simulink model "ssbdemof"  (Simulink 4.00)
settings: Solver=FixedStepDiscrete  SolverMode=SingleTasking  StartTime=0.0  StopTime=99999999  RelTol=1e-3  AbsTol=1e-6
libraries: dspsnks3 x2, dspsrcs3 x2, simulink3 x2, dspxfrm3 x1, dspindex x1
settings Model: CovMetricSettings=d  Creator=don  LastModifiedBy=asharma  SaveTime=off  SaveOutput=off  LimitDataPoints=off  IntegerOverflowMsg=none  RTWOptions=-aRollThreshold=2  ExtModeTrigMode=oneshot  ExtModeArmWhenConnect=off  BlockReductionOpt=off

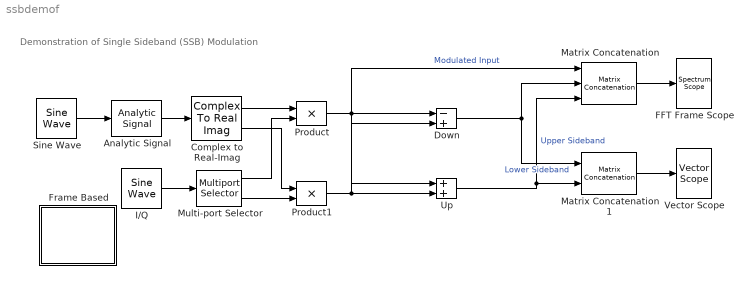
== system ssbdemof ==
  note: Demonstration of
      | Single Sideband (SSB)
      | Modulation
  Analytic Signal : dspxfrm3/Analytic Signal  N=100
  Complex to Real-Imag : ComplexToRealImag  Output=RealAndImag
  Down : Sum  Inputs=-+  SaturateOnIntegerOverflow=on
  FFT Frame Scope : dspsnks3/Spectrum Scope  ScopeProperties=on  Domain=Frequency  HorizSpan=1  UseBuffer=off  BufferSize=128  Overlap=64  inpFftLenInherit=off  FFTlength=64  numAvg=2  DisplayProperties=off  AxisGrid=on  Memory=off  FrameNumber=off  AxisLegend=on  AxisZoom=on  OpenScopeAtSimStart=on  OpenScopeImmediately=off  FigPos=[92 225 318 324]  AxisProperties=off  XUnits=rad/sec  XRange=[0...Fs/2]  InheritXIncr=on  XIncr=1  XLabel=Samples  YUnits=dB  YLabel=Magnitude, dB  LineProperties=off  LineColors=[0 0 0]|[1 0 1]|[0 0 1]
      settings: YMin=-111.54282150682  YMax=10.7226260336711
  Frame Based : Subsystem
      settings: OpenFcn=ssbdemo;  RTWFcnNameOpts=Auto  RTWFileNameOpts=Auto
      mask Display: disp('Sample-based\nVersion')
  I/Q : dspsrcs3/Sine Wave  Amplitude=1  Frequency=2  Phase=[0 pi/2]  SampleMode=Discrete  OutComplex=Real  CompMethod=Trigonometric Fcn  TableSize=Speed  SampleTime=0.1  SamplesPerFrame=64  ResetState=Restart at time zero
  Matrix Concatenation : simulink3/Signals & Systems/Matrix Concatenation  numInports=3  catMethod=Horizontal
  Matrix Concatenation1 : simulink3/Signals & Systems/Matrix Concatenation  numInports=2  catMethod=Horizontal
  Multi-port Selector : dspindex/Multiport Selector  rowsOrCols=Columns  idxCellArray={ 1, 2 }  idxErrMode=Clip Index
  Product : Product  Inputs=2  Multiplication=Element-wise(.*)  SaturateOnIntegerOverflow=on
  Product1 : Product  Inputs=2  Multiplication=Element-wise(.*)  SaturateOnIntegerOverflow=on
  Sine Wave : dspsrcs3/Sine Wave  Amplitude=1  Frequency=0.5  Phase=0  SampleMode=Discrete  OutComplex=Real  CompMethod=Trigonometric Fcn  TableSize=Speed  SampleTime=0.1  SamplesPerFrame=64  ResetState=Restart at time zero
  Up : Sum  Inputs=++  SaturateOnIntegerOverflow=on
  Vector Scope : dspsnks3/Vector Scope  ScopeProperties=on  Domain=Time  HorizSpan=1  DisplayProperties=off  AxisGrid=on  Memory=off  FrameNumber=on  AxisLegend=on  AxisZoom=on  OpenScopeAtSimStart=on  OpenScopeImmediately=off  FigPos=[425 221 457 327]  AxisProperties=off  XUnits=Hertz  XRange=[0...Fs/2]  InheritXIncr=on  XIncr=1  XLabel=Samples  YUnits=dB  YLabel=Amplitude  LineProperties=off  LineColors=[1 0 1]|[0 0 1]
      settings: YMin=-1.04989634553767  YMax=1.04996004090518
  wires:
  Sine Wave/1 -> Analytic Signal/1
  Analytic Signal/1 -> Complex to Real-Imag/1
  Product/1 -> Down/1, Up/1, Matrix Concatenation/1  "Modulated Input"
  Product1/1 -> Up/2, Down/2
  Complex to Real-Imag/2 -> Product1/1
  Multi-port Selector/2 -> Product1/2
  Complex to Real-Imag/1 -> Product/1
  Multi-port Selector/1 -> Product/2
  Down/1 -> Matrix Concatenation1/1, Matrix Concatenation/2  "Lower Sideband"
  Up/1 -> Matrix Concatenation/3, Matrix Concatenation1/2  "Upper Sideband"
  I/Q/1 -> Multi-port Selector/1
  Matrix Concatenation/1 -> FFT Frame Scope/1
  Matrix Concatenation1/1 -> Vector Scope/1

== system ssbdemof/Frame Based ==
